simulink model "ultra"  (R2020b)
settings: Solver=FixedStepDiscrete  StartTime=0.0  StopTime=10.0  FixedStep=0.0005  RelTol=1e-3  EnableMultiTasking=on
undefined symbols (not defined in the file): acc_calmax1, acc_calmax2, acc_calmin1, acc_calmin2, akemancanshu, bre, bre_calmax, bre_calmin, ecucoder_acal, I_AN01_5K1, I_AN03_5V, I_AN04_5V, kd, ki, kp, leftmax, O_SW06_HS1A, rightmax, T_add, T_del, tiaoshi, zhiling
libraries: ec5744lib x215, canmsglib x75, simulink x10
(part 6 of 7)

== matlab function ultra/转向自动标定/MATLAB Function1 ==
  data: model input; y output; status input
function y = fcn(model,status)
if (model==2)
    y=1;
else
    y=0;
end

== matlab function ultra/转向自动标定/转向自动标定/MATLAB Function ==
  data: biaozhi1 output
function biaozhi1  = fcn()
persistent i;
     % 初始化状态变量
    if isempty(i)
        i = 1;
    end

    if i>4
        biaozhi1=1;
    else
        biaozhi1=0;       
    end
i=i+1;
end

== matlab function ultra/转向自动标定/转向自动标定/MATLAB Function1 ==
  data: y1 output; y2 output; biaozhi2 output
function [y1,y2,biaozhi2] = fcn()
    persistent i;
     % 初始化状态变量
    if isempty(i)
        i = 1;
    end
    
    if i<4
        biaozhi2=1;
    else
        biaozhi2=0;
    end
    if mod(i, 2) == 0
        result = 1;
    else
        result = 0;
    end
    
    if result==0
        y1=6307883;
        y2=0;
    else
        y1=6307883;
        y2=128;
    end
    i=i+1;

== matlab function ultra/TOWORKSTATION/MATLAB Function ==
  data: u input; y output
function y = fcn(u)
if u~=0&&u~=9&&u~=2
    y=1;
else
    y=0;
end

== matlab function ultra/esc,ABS/Subsystem/MATLAB Function ==
  data: u input; y output; status input
function y = fcn(u,status)
y = u;
if status==5
    u=4500;
end

== matlab function ultra/run/analog_input/有人/Subsystem/MATLAB Function5 ==
  data: acc_fin_sig1 input; y output; acc_fin_sig2 input; bre_ori_sig input; bre input
function y = fcn(acc_fin_sig1, acc_fin_sig2,bre_ori_sig,bre)
if abs(acc_fin_sig1-acc_fin_sig2)>0.6
    y=0;
elseif acc_fin_sig2>0.5&&bre_ori_sig+bre==2
    y=0;
else
    y=acc_fin_sig1;
end

== matlab function ultra/esc,ABS/Subsystem/MATLAB Function1 ==
  data: u input; y output; status input
function y = fcn(u,status)
y = u;
if status==5
    u=4500;
end

== matlab function ultra/esc,ABS/Subsystem/MATLAB Function2 ==
  data: u input; y output; status input
function y = fcn(u,status)
y = u;
if status==5
    u=4500;
end

== matlab function ultra/esc,ABS/Subsystem/MATLAB Function3 ==
  data: u input; y output; status input
function y = fcn(u,status)
y = u;
if status==5
    u=4500;
end

== matlab function ultra/转向自动标定/转向自动标定/Subsystem/MATLAB Function ==
  data: steer output; y output; rm input; lm input; bianmaqi input; k output; d output
function [steer,y,k,d] = fcn(rm,lm,bianmaqi)
%使用前请将转向打到最左侧
lm=lm+3000;
rm=rm-3000;
k=0;
d=0;
  persistent i  A B;
     % 初始化状态变量
    if isempty(i)
        i = 0;
        A=zeros(120,1);
        B=zeros(120,1);
    end
 
    if i>20&&i<=140  
        j=i-20;
        delta=(rm-lm)/120;
        steer= lm+j*delta ;
        if (j>=1&&j<=120)
            B(j,1)=steer-delta;
            A(j,1)=bianmaqi;
        end
        
    else
      if i>=140
            N=length(A);
%             bb=0;
%             aa=0;
%             for l=1:120
%                 bbb=bb+B(l,1);
%                 aaa=aa+A(l,1);
%             end
%             bbar=bbb/120;
%             abar=aaa/120;
            k=(sum(B.*A)-N*mean(B)*mean(A))/(sum(A.^2)-N*mean(A)^2);
            d=mean(B)-k*mean(A);
%             steer=single(d);
        end
        steer=lm;
    end

    i=i+1;
  persistent time  a b;
     % 初始化状态变量
    if isempty(time)
        time = 0;
   
        a=5;
        b=10;
    end
    if mod(abs(time), 2) == 0
        result = 1;
    else
        result = 0;
    end
    if time<b&&result==0
    y=6;
 
    elseif time<b&&result==1
    y=15;
  
    elseif time>=b
        if result==1
            y=79;
        else
            y=63;
        end
    else
        y=6;
    end   
    time=time+1;
 
%     
%       persistent time1;
%      % 初始化状态变量
%     if isempty(time1)
%         time1 = 0;
%     end
%     if mod(time1, 2) == 0
%         result1 = 1;
%     else
%         result1 = 0;
%     end
%     if time1<2
%     y=6;
%  
%     elseif time1>=2&&time1<4
%     y=15;
%   
%     elseif time1>=4
%         if result1==1
%             y=79;
%         else
%             y=63;
%         end
%     else
%         y=6;
%     end   
%     time1=time1+1;
   
end

== matlab function ultra/run/analog_input/有人/Subsystem/Subsystem1/MATLAB Function ==
  data: u input; y output
function y = fcn(u)
if u==0
    y=0;
else
    y=1;
end

== matlab function ultra/run/MATLAB Function ==
  data: u input; y output; u1 input; model input
function y = fcn(u,u1,model)
if ((u>0.8&&model==0)||(u1>0.8))
    y = 1;
else
    y=0;
end

== matlab function ultra/run/LQR ==
  data: x input; y output
function y = fcn(x)
% A=[1 1;1 1];
% size(A,1);
% B=[1;1];
% P=size(B,2);
% ts=0.02;%离散时间的步长
% sys_d=c2d(ss(A,B),ts);%连续转离散系统函数，用于仿真代码
% x0=[1,1];%系统初始化
% x=x0;
% u0=0;
% u=u0;
% Q=[1 0 ;0 1];%系统权重
% S=[1 0;0 1];%终值权重
% R=0.1;%输入权重
% %定义系统运行步数
% k_steps = 100;
% %定义x._history雩矩阵,用于储存系统状态结果
% xhistory = zeros(n ,k_steps) ;
% %俘系统状态初始值赋值到x_history矩阵第一个位置
% xhistory (:,l)= x;
% %定义u_history需矩阵,用于储存系统输入结果,
% u_history = zeros(p,k_steps) ;
% %俘系统输入初始值赋值到u_history矩阵第一个位置
% u_history (:,1) = u;
% P_k = s;
% %计算最优反馈增益
% 
% 
% % 计算最优反馈增益
% for k = l : N
% % 计算F[N-k]
% F= inv(R+B'*P_k*B)*B'*P_k*A;
% 
% N= k_steps;
% P_k = s;
% % 计算最优反馈增益
% 
% P_k = (A-B*F)'*P_k*(A-B*F)+(F)'*R*(F)+Q;
% if k ==l
% F_N=F;
% else
% F_N=[F;F_N];
% end
% %仿真开始,建立for循环
% for k=l:k_steps
% u =-FN((k-1)*p+l:k*p ,:)*x;
% x= A*x+B*u ;
% %保存系统状态到预先定义矩阵的相应位置
% x_history(: ,k+l)=x;
% %保存系统输入到预先定义矩阵的相应位置
% u_history ( :,k)=u ;
% end
% 
% y=u;

== matlab function ultra/run/ctrl/Subsystem1/control_strategy/MPC ==
  data: X_K input; y output; Prediction input; A input; B input; Q input; R input; F input
function y = fcn(X_K,Prediction,A,B,Q,R,F)
    U_K(:,k) = Prediction;
    % 计算第k+1步时状态变量的值
%     X_K(:,k+1) = (A*X_K(:,k) + B*U_K(:,k))-0.17*A;
end

== matlab function ultra/run/ctrl/Subsystem1/control_strategy/限滑/MPC/MPC/MPC右后/MPC_function ==
  data: x_k input; u_k output; U_init input
function u_k= Prediction(x_k,U_init)
% 定义状态矩阵 A, n*n 矩阵
A = 0;
% 定义输入矩阵 B, n*p 矩阵
R=0.2032;
FN=2058;
K=6.89;
B = R/(FN*K);
p = size(B,2);
% 定义Q矩阵，n*n 矩阵
Q = 100;
% 定义F矩阵，n*n 矩阵
F = 100;
% 定义R矩阵，p*p 矩阵
R = 1;
% 定义迭代次数和学习率
maxIterations = 5;
learningRate = 0.3;
N=5;%预测区间
n=size(A,1); % A是n*n矩阵,得到n
p=size(B,2); % B是n*p矩阵,得到p
M=[eye(n);zeros(N*n,n)]; % 初始化M矩阵,M矩阵是(N+1)n*n的
D=[0.17;zeros(N*n,n)];
C=zeros((N+1)*n,N*p); % 初始化C矩阵,这一步令它有(N+1)n*NP个0

% 定义M和C
tmp=eye(n); % 定义一个n*n 的 I 矩阵
    for i=1:N % 循环,i从1到N
        rows =i*n+(1:n); %定义当前行数,从i*n开始，共n行
        C(rows,:)=[tmp*B,C(rows-n, 1:end-p)]; %将c矩阵填满
        tmp= A*tmp; %每一次将tmp左乘一次A
        M(rows,:)=tmp; %将M矩阵写满
         D(rows,:)=0.17;
    end
    % 定义Q_bar和R_bar
    Q_bar = kron(eye(N),Q);
    Q_bar = blkdiag(Q_bar,F);
    R_bar = kron(eye(N),R);
    % 计算G,E,H
    G=M'*Q_bar*M; % G: n*n
    E=C'*Q_bar*M; % E: NP*n
    H=C'*Q_bar*C+R_bar; % NP*NP
 J=(D'*Q_bar*C)';
 L=E*x_k+J;
 U = U_init*ones(N*p,1); % NP x 1
%  options = optimoptions('quadprog', 'Algorithm', 'active-set');
%  U_k = quadprog(H,L, [], [], [], [], 0*ones(5,1), 1100*ones(5,1), 100*ones(5,1), options);
    % 梯度下降法求解最优二次规划问题
    G=size(U,1);
    S=zeros(G*maxIterations,1);
    for i = 1:maxIterations
        % 计算目标函数的梯度
        gradient = 2*H*U + 2*L;
        % 更新变量 U，并保持在 [0, 1100] 范围内
        U = U - learningRate * gradient;
        U = max(U, 0);
        U = min(U, 1100);
        O=(i-1)*maxIterations+(1:maxIterations);
        S(O,1)=U;
    end

 u_k = S(1:p,1); % 取第一个结果
end

== matlab function ultra/run/ctrl/Subsystem1/control_strategy/E,H ==
  data: A input; E output; B input; Q input; R input; F input; N input; H output; J output
function [E,H,J] = MPC_Matrices(A,B,Q,R,F,N)
    n=size(A,1); % A是n*n矩阵,得到n
    p=size(B,2); % B是n*p矩阵,得到p
    M=[eye(n);zeros(N*n,n)]; % 初始化M矩阵,M矩阵是(N+1)n*n的,
                             % 它上面是n*n个"I",这一步先把下半部分写成0
    C=zeros((N+1)*n,N*p); % 初始化C矩阵,这一步令它有(N+1)n*NP个0
     D=zeros(1,N*p);
    % 定义M和C
    tmp=eye(n); % 定义一个n*n 的 I 矩阵
    % 更新Ｍ和C
    for i=1:N % 循环,i从1到N
        rows =i*n+(1:n); %定义当前行数,从i*n开始，共n行
        C(rows,:)=[tmp*B,C(rows-n, 1:end-p)]; %将c矩阵填满
        tmp= A*tmp; %每一次将tmp左乘一次A
        M(rows,:)=tmp; %将M矩阵写满
    end
    % 定义Q_bar和R_bar
    Q_bar = kron(eye(N),Q);
    Q_bar = blkdiag(Q_bar,F);
    R_bar = kron(eye(N),R);
    % 计算G,E,H
    G=M'*Q_bar*M; % G: n*n
    E=C'*Q_bar*M; % E: NP*n
    H=C'*Q_bar*C+R_bar; % NP*NP
for i=1:N % 循环,i从1到N
     D(i)= 0.17;
end
  J=C'*Q_bar*D'

== matlab function ultra/run/ctrl/Subsystem1/control_strategy/MATLAB Function2 ==
  data: A output; B output; Q output; R output; F output; N output; p output
function [A,B,Q,R,F,N,p] = fcn()
% 定义状态矩阵 A, n*n 矩阵
A = 0;
% 定义输入矩阵 B, n*p 矩阵
R=1;
FN=1;
K=6.89;
B = R/(FN*K);
p = size(B,2);
% 定义Q矩阵，n*n 矩阵
Q = 100;
% 定义F矩阵，n*n 矩阵
F = 100;
% 定义R矩阵，p*p 矩阵
R = 1;
%定义预测区间K
N = 5;

== matlab function ultra/run/ctrl/Subsystem1/control_strategy/差速/差速/LQR差速 ==
  data: yaw_error input; M output; yaw_rate input; J input
% function M = carLQRControl(yaw_error, yaw_rate,J)
%     % 赛车LQR控制器参数
%     Q = diag([1, 1]); % 状态误差权重矩阵
%     R = 0.1; % 控制输入权重
%     
%     % 定义车辆模型参数
%     % J转动惯量
%     
%     % 设计LQR增益矩阵 K
%     A = [0, 1; 0, 0];%输入为期望与实际横摆力矩差值和横摆角速度
%     B = [0; J];
%     K = lqr(A, B, Q, R);
%     
%     % 计算横摆力矩控制输入
%     M = -K* [yaw_error; yaw_rate];
function M = carLQRControl(yaw_error, yaw_rate,J)
    % 赛车LQR控制器参数
    Q = diag([1, 1]); % 状态误差权重矩阵
    R = 0.1; % 控制输入权重
    
    % 设计LQR增益矩阵 K
    A = [0, 1; 0, 0]; % 输入为期望与实际横摆力矩差值和横摆角速度
    B = [0; J];
    
    % 使用迭代法求解代数Riccati方程，计算LQR增益矩阵 K
    max_iterations = 20;
    tolerance = 1e-2;
    P = eye(size(A));
%     for i = 1:max_iterations
%         P_new = Q + A' * P * A - A' * P * B * (R + B' * P * B)^(-1) * B' * P * A;
%         if max(abs(P_new - P), [], 'all') < tolerance
%             P = P_new;
%             break;
%         end
%         P = P_new;
%   K = (R + B' * P * B)^(-1) * B' * P * A;
%     end
     % 计算LQR增益矩阵 

 
   for k = 1:max_iterations
        F = inv(R+B'*P*B)*B'*P*A;
        P_new = (A-B*F)'*P*(A-B*F)+(F)'*R*(F)+Q;
        if max(abs(P_new - P), [], 'all') < tolerance
             P= P_new;
             F = inv(R+B'*P*B)*B'*P*A;
            break;
        end
        P= P_new;
    end
    F_N=F; 
   
    % 计算横摆力矩控制输入
    M = -F_N * [yaw_error; yaw_rate];

end

== matlab function ultra/run/ctrl/Subsystem1/control_strategy/限滑/MPC/MPC/MPC左后/MPC_function ==
  data: x_k input; u_k output; U_init input
function u_k= Prediction(x_k,U_init)
% 定义状态矩阵 A, n*n 矩阵
A = 0;
% 定义输入矩阵 B, n*p 矩阵
R=0.2032;
FN=2058;
K=6.89;
B = R/(FN*K);
p = size(B,2);
% 定义Q矩阵，n*n 矩阵
Q = 100;
% 定义F矩阵，n*n 矩阵
F = 100;
% 定义R矩阵，p*p 矩阵
R = 1;
% 定义迭代次数和学习率
maxIterations = 5;
learningRate = 0.3;
N=5;%预测区间
n=size(A,1); % A是n*n矩阵,得到n
p=size(B,2); % B是n*p矩阵,得到p
M=[eye(n);zeros(N*n,n)]; % 初始化M矩阵,M矩阵是(N+1)n*n的
D=[0.17;zeros(N*n,n)];
C=zeros((N+1)*n,N*p); % 初始化C矩阵,这一步令它有(N+1)n*NP个0

% 定义M和C
tmp=eye(n); % 定义一个n*n 的 I 矩阵
    for i=1:N % 循环,i从1到N
        rows =i*n+(1:n); %定义当前行数,从i*n开始，共n行
        C(rows,:)=[tmp*B,C(rows-n, 1:end-p)]; %将c矩阵填满
        tmp= A*tmp; %每一次将tmp左乘一次A
        M(rows,:)=tmp; %将M矩阵写满
         D(rows,:)=0.17;
    end
    % 定义Q_bar和R_bar
    Q_bar = kron(eye(N),Q);
    Q_bar = blkdiag(Q_bar,F);
    R_bar = kron(eye(N),R);
    % 计算G,E,H
    G=M'*Q_bar*M; % G: n*n
    E=C'*Q_bar*M; % E: NP*n
    H=C'*Q_bar*C+R_bar; % NP*NP
 J=(D'*Q_bar*C)';
 L=E*x_k+J;
 U = U_init*ones(N*p,1); % NP x 1
%  options = optimoptions('quadprog', 'Algorithm', 'active-set');
%  U_k = quadprog(H,L, [], [], [], [], 0*ones(5,1), 1100*ones(5,1), 100*ones(5,1), options);
    % 梯度下降法求解最优二次规划问题
    G=size(U,1);
    S=zeros(G*maxIterations,1);
    for i = 1:maxIterations
        % 计算目标函数的梯度
        gradient = 2*H*U + 2*L;
        % 更新变量 U，并保持在 [0, 1100] 范围内
        U = U - learningRate * gradient;
        U = max(U, 0);
        U = min(U, 1100);
        O=(i-1)*maxIterations+(1:maxIterations);
        S(O,1)=U;
    end

 u_k = S(1:p,1); % 取第一个结果
end

== matlab function ultra/run/ctrl/Subsystem1/control_strategy/限滑/MPC/MPC/MPC右前/MPC_function ==
  data: x_k input; u_k output; U_init input
function u_k= Prediction(x_k,U_init)
% 定义状态矩阵 A, n*n 矩阵
A = 0;
% 定义输入矩阵 B, n*p 矩阵
R=0.2032;
FN=2058;
K=6.89;
B = R/(FN*K);
p = size(B,2);
% 定义Q矩阵，n*n 矩阵
Q = 100;
% 定义F矩阵，n*n 矩阵
F = 100;
% 定义R矩阵，p*p 矩阵
R = 1;
% 定义迭代次数和学习率
maxIterations = 5;
learningRate = 0.3;
N=5;%预测区间
n=size(A,1); % A是n*n矩阵,得到n
p=size(B,2); % B是n*p矩阵,得到p
M=[eye(n);zeros(N*n,n)]; % 初始化M矩阵,M矩阵是(N+1)n*n的
D=[0.17;zeros(N*n,n)];
C=zeros((N+1)*n,N*p); % 初始化C矩阵,这一步令它有(N+1)n*NP个0

% 定义M和C
tmp=eye(n); % 定义一个n*n 的 I 矩阵
    for i=1:N % 循环,i从1到N
        rows =i*n+(1:n); %定义当前行数,从i*n开始，共n行
        C(rows,:)=[tmp*B,C(rows-n, 1:end-p)]; %将c矩阵填满
        tmp= A*tmp; %每一次将tmp左乘一次A
        M(rows,:)=tmp; %将M矩阵写满
         D(rows,:)=0.17;
    end
    % 定义Q_bar和R_bar
    Q_bar = kron(eye(N),Q);
    Q_bar = blkdiag(Q_bar,F);
    R_bar = kron(eye(N),R);
    % 计算G,E,H
    G=M'*Q_bar*M; % G: n*n
    E=C'*Q_bar*M; % E: NP*n
    H=C'*Q_bar*C+R_bar; % NP*NP
 J=(D'*Q_bar*C)';
 L=E*x_k+J;
 U = U_init*ones(N*p,1); % NP x 1
%  options = optimoptions('quadprog', 'Algorithm', 'active-set');
%  U_k = quadprog(H,L, [], [], [], [], 0*ones(5,1), 1100*ones(5,1), 100*ones(5,1), options);
    % 梯度下降法求解最优二次规划问题
    G=size(U,1);
    S=zeros(G*maxIterations,1);
    for i = 1:maxIterations
        % 计算目标函数的梯度
        gradient = 2*H*U + 2*L;
        % 更新变量 U，并保持在 [0, 1100] 范围内
        U = U - learningRate * gradient;
        U = max(U, 0);
        U = min(U, 1100);
        O=(i-1)*maxIterations+(1:maxIterations);
        S(O,1)=U;
    end

 u_k = S(1:p,1); % 取第一个结果
end

== matlab function ultra/run/ctrl/Subsystem1/control_strategy/限滑/MPC/MPC/MPC左前/MPC_function ==
  data: x_k input; u_k output; U_init input
function u_k= Prediction(x_k,U_init)
% 定义状态矩阵 A, n*n 矩阵
A = 0;
% 定义输入矩阵 B, n*p 矩阵
R=0.2032;
FN=2058;
K=6.89;
B = R/(FN*K);
p = size(B,2);
% 定义Q矩阵，n*n 矩阵
Q = 100;
% 定义F矩阵，n*n 矩阵
F = 100;
% 定义R矩阵，p*p 矩阵
R = 1;
% 定义迭代次数和学习率
maxIterations = 5;
learningRate = 0.3;
N=5;%预测区间
n=size(A,1); % A是n*n矩阵,得到n
p=size(B,2); % B是n*p矩阵,得到p
M=[eye(n);zeros(N*n,n)]; % 初始化M矩阵,M矩阵是(N+1)n*n的
D=[0.17;zeros(N*n,n)];
C=zeros((N+1)*n,N*p); % 初始化C矩阵,这一步令它有(N+1)n*NP个0

% 定义M和C
tmp=eye(n); % 定义一个n*n 的 I 矩阵
    for i=1:N % 循环,i从1到N
        rows =i*n+(1:n); %定义当前行数,从i*n开始，共n行
        C(rows,:)=[tmp*B,C(rows-n, 1:end-p)]; %将c矩阵填满
        tmp= A*tmp; %每一次将tmp左乘一次A
        M(rows,:)=tmp; %将M矩阵写满
         D(rows,:)=0.17;
    end
    % 定义Q_bar和R_bar
    Q_bar = kron(eye(N),Q);
    Q_bar = blkdiag(Q_bar,F);
    R_bar = kron(eye(N),R);
    % 计算G,E,H
    G=M'*Q_bar*M; % G: n*n
    E=C'*Q_bar*M; % E: NP*n
    H=C'*Q_bar*C+R_bar; % NP*NP
 J=(D'*Q_bar*C)';
 L=E*x_k+J;
 U = U_init*ones(N*p,1); % NP x 1
%  options = optimoptions('quadprog', 'Algorithm', 'active-set');
%  U_k = quadprog(H,L, [], [], [], [], 0*ones(5,1), 1100*ones(5,1), 100*ones(5,1), options);
    % 梯度下降法求解最优二次规划问题
    G=size(U,1);
    S=zeros(G*maxIterations,1);
    for i = 1:maxIterations
        % 计算目标函数的梯度
        gradient = 2*H*U + 2*L;
        % 更新变量 U，并保持在 [0, 1100] 范围内
        U = U - learningRate * gradient;
        U = max(U, 0);
        U = min(U, 1100);
        O=(i-1)*maxIterations+(1:maxIterations);
        S(O,1)=U;
    end

 u_k = S(1:p,1); % 取第一个结果
end

== matlab function ultra/run/ctrl/Subsystem1/control_strategy/限滑/PID限滑/pid限滑与ABS ==
  data: slip input; throttle output; slip_ratio_limit input; brake output; u input
function [throttle, brake] = carPIDWithSlipControl(slip, slip_ratio_limit,u)
    % 赛车PID控制器参数
    kp = 0.2;
    ki = 0.1;
    kd = 0.01;
    
    % 状态变量
    persistent integral previous_error i
    
    % 初始化状态变量
    if isempty(integral)
        integral = 0;
        previous_error = 0;
        i=0;
    end
    
    % PID控制器计算
    error = 0.2 - slip;
    integral = integral + error*0.02;
    derivative = (error - previous_error)/0.02;
    
   k = kp * error + ki * integral + kd * derivative;
    if i<100
    
        output = u+k*u;
        if output>2000
            output=2000;
        end
    else
        output=u;
    end
    % 根据滑移率限制输出
  
    if slip > slip_ratio_limit
        brake = 0;%output;
        throttle = 0;
    else
        brake = 0;
        throttle = output;
    end
    
    % 保存上一个误差用于下次计算
    previous_error = error;

    i=i+1;
end

== matlab function ultra/run/analog_input/无人意图转译/无人/Subsystem1/MATLAB Function3 ==
  data: u input; y1 output; y2 output; v input; vd input; ade input; adede input; adedede input
function [y1,y2] = fcn(u,v,vd,ade,adede,adedede)
persistent i
    if isempty(i)
       
        i=0;
    end
dota=(u-i);
if v-vd>5
    u=0;
end
if u>=0
    if dota>1
    y1=(u+i+ade+adede+adedede)/5;
    else
    y1=u;
    end
    y2=0;
else
    y1=0;
    y2=u;
end

if u<0
    y2=u;
end
i=u;
end

== matlab function ultra/run/analog_input/无人意图转译/无人/Subsystem1/Subsystem/pid_function/integral ==
  data: u input; output output; a input
function output = fcn(u,a)
    % 赛车PID控制器参数
    kp = 0;
    ki = 0;
    kd = 0;
    
    % 状态变量
    persistent integral previous_error i
    
    % 初始化状态变量
    if isempty(integral)
        integral = 0;
        previous_error = 0;
        i=0;
    end
        if i>50
            i=0;
            ki = 0;
            kd = 0;
        end
    % PID控制器计算
    error = u;
%     integral = integral + error*0.02;
    derivative = (error - previous_error)/0.02;
    integral =0;
    if error<0.1
        ki=0;
    end
    output = kp * error + ki * integral + kd * derivative;
    
   if a==0
       output=0;
   end
    % 保存上一个误差用于下次计算
    previous_error = error;
    i=i+1
end

== matlab function ultra/run/analog_input/有人/Subsystem/MATLAB Function1 ==
  data: u input; y output; min input; max input
function y = fcn(u,min,max)
% 
% y = (double(u)-min-1270)/(max-min+2980-1270);
% y=0;
y=u;

== matlab function ultra/run/analog_input/无人意图转译/无人/Subsystem1/计算四轮各自制动力/MATLAB Function ==
  data: u input; y1 output; y2 output; y3 output; y4 output; deltaM input
function [y1,y2,y3,y4] = fcn(u,deltaM)


deltaM=0;
B=1.17;%轮距,前轮1.18后轮1.16
F1=1050;
F2=1050;%前后轮载荷，瞎设的，合并后引入
%a1 a2 b1 b2分别是左前轮制动力，右前轮制动力，左后轮制动力，右后轮制动力 方程： a1+a2+b1+b2==u/r;(a1+a2)/F1==(b1+b2)/F2;B*(a1-a2)/(2*F1)==B*(b1-b2)/(2*F2);(a1-a2)*B/2+(b1-b2)*B/2==deltaM;
b1=F2*u/(2*(F1+F2))+F2*deltaM/(F1*B+F2*B);
b2=F2*u/(2*(F1+F2))-F2*deltaM/(F1*B+F2*B);
a1=u/2-F2*u/(2*(F1+F2))+F1*deltaM/(F1*B+F2*B);
a2=u/2-F2*u/(2*(F1+F2))-F1*deltaM/(F1*B+F2*B);
y1=a1;
y2=a2;
y3=b1;
y4=b2;

== matlab function ultra/run/analog_input/无人意图转译/无人/Subsystem1/计算油压 ==
  data: y1 input; p1 output; y2 input; y3 input; y4 input; p2 output; p3 output; p4 output; zuoqian input; youqian input; zuohou input; youhou input; error input
function [p1,p2,p3,p4]= fcn(y1,y2,y3,y4,zuoqian,youqian,zuohou,youhou,error)
S=0.000491;
%p1 p2 p3 p4分别是左前、右前、左后、右后油压
p1=y1/(0.8*S)/1000*1.2;
p2=y2/(0.8*S)/1000*1.2;
p3=y3/(0.4*S)/1000*0.8;
p4=y4/(0.4*S)/1000*0.8;
    % 状态变量
    persistent  i1 i2 i3 i4 pp1 pp2 pp3 pp4
    
    % 初始化状态变量
    if isempty(i1)
        i1=0;
        i2=0;
        i3=0;
        i4=0;
        pp1=0;
        pp2=0;
        pp3=0;
        pp4=0;
    end
if abs(error)>0.6
    if p1>500||i1>0
        i1=i1+1;
        if p1<pp1
            if pp1-zuoqian>300
                p1=pp1-20;
            end
        end
    end
    if i1>49||abs(p1-zuoqian)<200
        i1=0;
    end
    if p2>500||i2>0
        i2=i2+1;
        if p2<pp2
            if pp2-youqian>300
                p2=pp2-20;
            end
        end
    end
    if i2>49||abs(p2-youqian)<200
        i2=0;
    end
    if p3>500||i3>0
        i3=i3+1;
        if p3<pp3
            if pp3-zuohou>300
                p3=pp3-20;
            end
        end
    end
    if i3>49||abs(p3-zuohou)<200
        i3=0;
    end
    if p4>500||i4>0
        i4=i4+1;
        if p4<pp4
            if pp4-youhou>300
                p4=pp4-20;
            end
        end
    end
    if i4>49||abs(p4-youhou)<200
        i4=0;
    end
end
 if error>0
     p1=0;
     p2=0;
     p3=0;
     p4=0;
 end
    pp1=p1;
    pp2=p2;
    pp3=p3;
    pp4=p4;
 
% if p1<0
%     p1=0;
%     end
% if p2<0
%     p2=0;
%     end
% if p3<0
%     p3=0;
%     end
% if p4<0
%     p4=0;
% end

== matlab function ultra/run/analog_input/无人意图转译/无人/MATLAB Function3 ==
  data: u input; y output
function y = fcn(u)
if u~=0
    y = 1;
else
    y=0;
end

== matlab function ultra/run/analog_input/无人意图转译/计算期望扭矩 ==
  data: u input; y output; canok input
function y = fcn(u,canok)

y = u*230*86.08;
if y>2000
    y=2000;
end
if canok==0
    y=0;
end

== matlab function ultra/run/analog_input/无人意图转译/无人/Subsystem1/id ==
  data: u input; output output
function output = fcn(u)
    % 赛车ID控制器参数
  
    ki = 0;
    kd = 0;
    
    % 状态变量
    persistent integral previous_error i
    
    % 初始化状态变量
    if isempty(integral)
        integral = 0;
        previous_error = 0;
        i=0;
    end
    if i>50
        i=0;
        ki = 0;
        kd = 0;
    end
    % PID控制器计算
    error = u;
    integral = integral + error*0.02;
    derivative = (error - previous_error)/0.02;
     if error<0.1
        ki=0;
    end
    output =  ki * integral + kd * derivative;
    if error<0.1
        ki=0;
    end
  
    % 保存上一个误差用于下次计算
    previous_error = error;
    if output>10
        output=0;
    end
    i=i+1;
end

== matlab function ultra/RX/lcu——receive/Subsystem1/Subsystem/MATLAB Function ==
  data: m input; y1 output; y2 output; y3 output
function [y1,y2,y3] = fcn(m)
V=zeros(1,3);
a=2;i=3;
while i>0
    V(1,i)=mod(m,a);
    m=fix(m/2);
    i=i-1;
end  
y1 = V(1,3);
y2=V(1,2);
y3=V(1,1);
end

== matlab function ultra/RX/lcu——receive/Subsystem1/Subsystem/MATLAB Function1 ==
  data: u input; y output
function y = fcn(u)
if u==7
    y = 1;
else
    y=0;
end
end

== matlab function ultra/run/ctrl/Subsystem1/control_strategy/差速/差速/期望横摆力矩计算 ==
  data: delta input; Mz output; Vx input; ax input
function Mz = calculateYawMoment(delta,  Vx, ax)
    % 输入参数：
    % delta: 前轮转角 (rad)
    % Vx: 车辆速度 (m/s)
    % ax: 侧向加速度 (m/s^2)
    m=210;%: 车辆质量 (kg)
     lf=0.765;%: 前轴到重心的距离 (m)
     lr=0.765;%: 后轴到重心的距离 (m)
    
    % 轮胎侧向力估计，这里使用一个简化的线性模型
    Fy = ax * (lr * m * 9.81) / (lf + lr);
    delta=delta*pi/180
    % 计算期望的横摆力矩
    Mz = lf * Fy * cos(delta);
end

== matlab function ultra/run/ctrl/Subsystem1/control_strategy/限滑/PID限滑/pid限滑与ABS1 ==
  data: slip input; throttle output; slip_ratio_limit input; brake output; u input
function [throttle, brake] = carPIDWithSlipControl(slip, slip_ratio_limit,u)
    % 赛车PID控制器参数
    kp = 0.2;
    ki = 0.1;
    kd = 0.01;
    
    % 状态变量
    persistent integral previous_error i
    
    % 初始化状态变量
    if isempty(integral)
        integral = 0;
        previous_error = 0;
        i=0;
    end
    
    % PID控制器计算
    error = 0.2 - slip;
    integral = integral + error*0.02;
    derivative = (error - previous_error)/0.02;
    
   k = kp * error + ki * integral + kd * derivative;
    if i<100
    
        output = u+k*u;
        if output>2000
            output=2000;
        end
    else
        output=u;
    end
    % 根据滑移率限制输出
  
    if slip > slip_ratio_limit
        brake = 0;%output;
        throttle = 0;
    else
        brake = 0;
        throttle = output;
    end
    
    % 保存上一个误差用于下次计算
    previous_error = error;
    i=i+1;
end

== matlab function ultra/run/analog_input/有人/Subsystem/MATLAB Function ==
  data: u input; y output; min input; max input
function y = fcn(u,min,max)

y = (double(u)-min-4765)/(-min+max-4765+4900);

== matlab function ultra/run/ctrl/Subsystem1/control_strategy/限滑/PID限滑/pid限滑与ABS2 ==
  data: slip input; throttle output; slip_ratio_limit input; brake output; u input
function [throttle, brake] = carPIDWithSlipControl(slip, slip_ratio_limit,u)
    % 赛车PID控制器参数
    kp = 0.2;
    ki = 0.1;
    kd = 0.01;
    
    % 状态变量
    persistent integral previous_error i
    
    % 初始化状态变量
    if isempty(integral)
        integral = 0;
        previous_error = 0;
        i=0;
    end
    
    % PID控制器计算
    error = 0.2 - slip;
    integral = integral + error*0.02;
    derivative = (error - previous_error)/0.02;
   k = kp * error + ki * integral + kd * derivative;
    if i<100
    
        output = u+k*u;
        if output>2000
            output=2000;
        end
    else
        output=u;
    end
    % 根据滑移率限制输出
  
    if slip > slip_ratio_limit
        brake = 0;%output;
        throttle = 0;
    else
        brake = 0;
        throttle = output;
    end
    
    % 保存上一个误差用于下次计算
    previous_error = error;
    i=i+1;
end

== matlab function ultra/run/ctrl/Subsystem1/control_strategy/限滑/PID限滑/pid限滑与ABS3 ==
  data: slip input; throttle output; slip_ratio_limit input; brake output; u input
function [throttle, brake] = carPIDWithSlipControl(slip, slip_ratio_limit,u)
    % 赛车PID控制器参数
    kp = 0.2;
    ki = 0.1;
    kd = 0.01;
    
    % 状态变量
    persistent integral previous_error i
    
    % 初始化状态变量
    if isempty(integral)
        integral = 0;
        previous_error = 0;
        i=0;
    end
    
    % PID控制器计算
    error = 0.2 - slip;
    integral = integral + error*0.02;
    derivative = (error - previous_error)/0.02;
    
   k = kp * error + ki * integral + kd * derivative;
    if i<100
    
        output = u+k*u;
        if output>2000
            output=2000;
        end
    else
        output=u;
    end
    % 根据滑移率限制输出
  
    if slip > slip_ratio_limit
        brake =0;% output;
        throttle = 0;
    else
        brake = 0;
        throttle = output;
    end
    
    % 保存上一个误差用于下次计算
    previous_error = error;
    i=i+1;
end

== matlab function ultra/run/ctrl/Subsystem1/control_strategy/MATLAB Function1 ==
  data: y output; angle input
function y = fcn(angle)
if angle>30||angle<-30%4650000,4870000,4741002
    y=1;
else
    y = 0;
end

== matlab function ultra/run/ctrl/Subsystem1/control_strategy/限滑/Subsystem1/MATLAB Function2 ==
  data: u input; y output; mpc input; pid input; slip input; model input
function y = fcn(u,mpc,pid,slip,model)
if slip>0.8&&model~=6
    y=pid;
elseif slip>0.165&&slip<0.17
        y=mpc;
else
        y=u;
end
end

== matlab function ultra/run/ctrl/Subsystem1/control_strategy/限滑/Subsystem1/MATLAB Function3 ==
  data: u input; y output; mpc input; pid input; slip input; model input
function y = fcn(u,mpc,pid,slip,model)
if slip>0.8&&model~=6
    y=pid;
elseif slip>0.169&&slip<0.17
        y=mpc;
else
        y=u;
end
end

== matlab function ultra/run/ctrl/Subsystem1/control_strategy/限滑/Subsystem1/MATLAB Function4 ==
  data: u input; y output; mpc input; pid input; slip input; model input
function y = fcn(u,mpc,pid,slip,model)
if slip>0.8&&model~=6
    y=pid;
elseif slip>0.165&&slip<0.17
        y=mpc;
else
        y=u;
end
end

== matlab function ultra/run/ctrl/Subsystem1/control_strategy/限滑/Subsystem1/MATLAB Function5 ==
  data: u input; y output; mpc input; pid input; slip input; model input
function y = fcn(u,mpc,pid,slip,model)
if slip>0.8&&model~=6
    y=pid;
elseif slip>0.165&&slip<0.17
        y=mpc;
else
        y=u;
end
end

== matlab function ultra/run/ctrl/Subsystem1/control_strategy/差速/MATLAB Function3 ==
  data: u input; youhou output; M input; youqian output; zuohou output; zuoqian output
function [youhou,youqian,zuohou,zuoqian] = fcn(u,M)
% U=4*u;
r=0.2032;%轮半径
B1=1.18;%左右轮距
B2=1.16;
youqian=M*r/(2*B2)+u;
youhou=youqian;
zuoqian=-M*r/(2*B1)+u;
zuohou=zuoqian;
end

== matlab function ultra/run/ctrl/Subsystem1/control_strategy/Subsystem/defuzzification ==
  data: dnb input; delta output; dns input; do input; dps input; dpb input; d1 input; d2 input; d3 input
function delta = fcn(dnb,dns,do,dps,dpb, d1,d2,d3)
delta = dnb*d1/3 + dns*d1 + do*d2 + dps*d3 + dpb*(1-d3/3);
end

== matlab function ultra/run/analog_input/有人/Subsystem/MATLAB Function2 ==
  data: u input; y output; min input; max input
function y = fcn(u,min,max)

y = (double(u)-min-4670)/(-min+0.01+max-4670+4550);

== matlab function ultra/run/ctrl/Subsystem1/control_strategy/Subsystem/α sets ==
  data: alpha input; as output; am output; ab output; a1 input; a2 input
function [as,am,ab] = fcn(alpha, a1, a2)
if alpha < a1
    as = 1-(alpha/a1);
    am = alpha/a1;
    ab = 0;
elseif alpha < a2
    as = 0; 
    am = 1-(alpha-a1)/(a2-a1);
    ab = (alpha-a1)/(a2-a1);
else
    as = 0;
    am = 0;
    ab = 1;
end

== matlab function ultra/run/ctrl/Subsystem1/control_strategy/Subsystem/β sets ==
  data: beta input; bnb output; bns output; bo output; b1 input; b2 input; bps output; bpb output; b3 input
function [bnb,bns,bo,bps,bpb] = fcn(beta, b1, b2, b3)
if beta < b1
    bnb = 1-(beta+1)/(b1+1);
    bns = (beta+1)/(b1+1);
    bo  = 0;
    bps = 0;
    bpb = 0;
elseif beta < b2
    bnb = 0; 
    bns = 1-(beta-b1)/(b2-b1);
    bo = (beta-b1)/(b2-b1);
    bps = 0;
    bpb = 0;
elseif beta < b3
    bnb = 0;
    bns = 0;
    bo  = 1-(beta-b2)/(b3-b2);
    bps = (beta-b2)/(b3-b2);
    bpb = 0;
else
    bnb = 0;
    bns = 0;
    bo  = 0;
    bps = 1-(beta-b3)/(1-b3);
    bpb = (beta-b3)/(1-b3);
end

== matlab function ultra/run/ctrl/Subsystem1/control_strategy/限滑/PID限滑/计算油压 ==
  data: y1 input; p1 output; y2 input; y3 input; y4 input; p2 output; p3 output; p4 output
function [p1,p2,p3,p4]= fcn(y1,y2,y3,y4)
S=0.000491;
%p1 p2 p3 p4分别是左前、右前、左后、右后油压
p1=y1/(0.8*S)/1000;
p2=y2/(0.8*S)/1000;
p3=y3/(0.4*S)/1000;
p4=y4/(0.4*S)/1000;
% if p1<0
%     p1=0;
%     end
% if p2<0
%     p2=0;
%     end
% if p3<0
%     p3=0;
%     end
% if p4<0
%     p4=0;
% end

== matlab function ultra/TX控制器/速度/184左前/MATLAB Function1 ==
  data: v input; T output; a input
function T = fcn(v,a)
% if a>5
%     y = u;
% elseif a>3&&a<5
%     y=1200;
% else
%     y=800;
% end

if v<6000*1.88e-3
    T=2100;
elseif v>11000*1.88e-3
    T=800;
else
    T=1100;
end

== matlab function ultra/TX控制器/速度/188右后/MATLAB Function1 ==
  data: v input; T output; a input
function T = fcn(v,a)
% if a>5
%     y = u;
% elseif a>3&&a<5
%     y=1200;
% else
%     y=800;
% end

if v<6000*1.88e-3
    T=2100;
elseif v>11000*1.88e-3
    T=800;
else
    T=1100;
end

== matlab function ultra/RX/转向——receive1/Subsystem3/Subsystem/MATLAB Function ==
  data: u input; y output
function y = fcn(u)
y =   0.0003056 *u-208.4  ;
if u==683198
    y=0;
end

== matlab function ultra/run/analog_input/MATLAB Function2 ==
  data: u input; y output; canok input
function y = fcn(u,canok)
if u==0%&&canok==1
    y=1;
else
    y=0;
end

== matlab function ultra/run/ctrl/Subsystem1/control_strategy/差速/差速/MATLAB Function ==
  data: u input; y output
function y = fcn(u)

y = u;

== matlab function ultra/run/MATLAB Function2 ==
  data: u input; y output
function y = fcn(u)
if u>500
    y=1;
else
    y=0;
end
if u>1800
    y=2;
end

== matlab function ultra/run/analog_input/有人/Subsystem1/MATLAB Function1 ==
  data: T input; TP output
function TP= fcn(T)
if T<10
    TP=0;
else
    TP=T;
end

== matlab function ultra/run/analog_input/MATLAB Function ==
  data: u input; y output
function y = fcn(u)
if u==9
    y=1;
else
    y=0;
end

== matlab function ultra/run/analog_input/MATLAB Function1 ==
  data: u input; y output; a input
function y = fcn(u,a)
if u==1
    y=15;%%无人规则缓慢转轮
else
    y=a;
end
end

== matlab function ultra/run/analog_input/MATLAB Function3 ==
  data: u input; y output; canok input; workstation input; v input
function y = fcn(u,canok,workstation,v)
if u~=0%%||canok==0
    y=1;
else
    y=0;
end
% if canok==0
%     y=0;
% end
%  if workstation<=0.1
%      y=0;
%  end
%  if v<0.5||v>18
%      y=0;
%  end

== matlab function ultra/run/analog_input/有人/Subsystem1/MATLAB Function ==
  data: v input; T output
function T = fcn(v)
%#codegen
if v<6000*1.88e-3
    T=2100;
elseif v>11000*1.88e-3
    T=800;
else
    T=1100;
end

== matlab function ultra/run/ctrl/Subsystem1/control_strategy/限滑/MPC/MPC/MATLAB Function ==
  data: u input; y output
function y = fcn(u)
if u>=0.169&&u<=0.17
    y=1;
else
    y=0;
end

end

== matlab function ultra/run/ctrl/Subsystem1/control_strategy/限滑/MPC/MPC/MATLAB Function1 ==
  data: u input; y output
function y = fcn(u)
if u>=0.169&&u<=0.17
    y=1;
else
    y=0;
end

end

== matlab function ultra/run/ctrl/Subsystem1/control_strategy/限滑/MPC/MPC/MATLAB Function2 ==
  data: u input; y output
function y = fcn(u)

if u>=0.169&&u<=0.17
    y=1;
else
    y=0;
end

end

== matlab function ultra/run/ctrl/Subsystem1/control_strategy/限滑/MPC/MPC/MATLAB Function3 ==
  data: u input; y output
function y = fcn(u)

if u>=0.169&&u<=0.17
    y=1;
else
    y=0;
end

end

== matlab function ultra/run/ctrl/Subsystem1/control_strategy/MATLAB Function3 ==
  data: y output; angle input
function y = fcn(angle)
if angle>10||angle<-10%4650000,4870000,4741002
    y=1;
else
    y = 0;
end

== matlab function ultra/TX控制器/速度/189左后/MATLAB Function1 ==
  data: v input; T output; a input
function T = fcn(v,a)
% if a>5
%     y = u;
% elseif a>3&&a<5
%     y=1200;
% else
%     y=800;
% end

if v<6000*1.88e-3
    T=2100;
elseif v>11000*1.88e-3
    T=800;
else
    T=1100;
end

== matlab function ultra/RX/lcu——receive/MATLAB Function ==
  data: m input; enable_185 output; enable_185_1 output; enable_188 output; enable_188_1 output; enable_184 output; enable_184_1 output; enable_189 output; enable_189_1 output
%八位无符号数
function [enable_185,enable_185_1,enable_188,enable_188_1,enable_184,enable_184_1,enable_189,enable_189_1] = ErJinZhi(m)
V=zeros(1,8);
a=2;i=8;
while i>0
    V(1,i)=mod(m,a);
    m=fix(m/2);
    i=i-1;
end    
enable_185=V(1,1);%右前
enable_185_1=V(1,2);
enable_188=V(1,3);%右后
enable_188_1=V(1,4);
enable_184=V(1,5);
enable_184_1=V(1,6);%左前
enable_189=V(1,7);
enable_189_1=V(1,8);%左后
end

== matlab function ultra/esc,ABS/MATLAB Function ==
  data: u input; y output
function y = fcn(u)
if u~=0&&u~=9&&u~=2
    y=1;
else
    y=0;
end

== matlab function ultra/run/analog_input/MATLAB Function4 ==
  data: u input; y output; a input
function y = fcn(u,a)
if u==5
    y=0;
else
    y=a;
end
end

== matlab function ultra/RX/工作站/Subsystem3/Subsystem/MATLAB Function ==
  data: u input; y output; CANOK_20 input
function y = fcn(u,CANOK_20)
if CANOK_20==0
    y=0;
else
    y=u;
end

== matlab function ultra/run/analog_input/MATLAB Function5 ==
  data: u input; y output; model input; y6 output
function [y,y6] = fcn(u,model)
if model==8
    y = 0;
    y6=u;
else
    y=u;
    y6=0;
end
if y~=0&&y6~=0
    y=0;
    y6=0;
end
    
end

== matlab function ultra/RX/工作站/Subsystem3/Subsystem/MATLAB Function1 ==
  data: u input; y output; CANOK_20 input
function y = fcn(u,CANOK_20)
% if CANOK_20==0
%     y=0;
% else
    y=u;
% end

== matlab function ultra/无人TX/MATLAB Function1 ==
  data: model input; y output; status input
function y = fcn(model,status)
if (model==1||model==3||model==4||model==6||model==7||model==8)&&(status==3||status==4||status==5)
    y=1;
else
    y=0;
end
if model==8
    y=1;
else
    y=y;
end

== matlab function ultra/无人TX/转向换算/MATLAB Function ==
  data: biaozhi1 output; baocuo input
function biaozhi1  = fcn(baocuo)
persistent i;
     % 初始化状态变量
    if isempty(i)
        i = 1;
    end
    if baocuo==1
        i=1;
    end
    if i>4
        biaozhi1=1;
    else
        biaozhi1=0;       
    end
i=i+1;
end

== matlab function ultra/无人TX/转向换算/Subsystem/MATLAB Function ==
  data: steer output; y output; x input; canok input; baocuo input; k input; d input; rm input; lm input
function [steer,y] = fcn(x,canok,baocuo,k,d,rm,lm)
  persistent i previoussteer;
     % 初始化状态变量
     rm=rm-3000;
     lm=lm+3000;
    if isempty(i)
        i = 0;
    end
    if isempty(previoussteer)
        previoussteer= d;
    end
    if i>0.2     
        steer= k *x+d ;
%         if x==0
%             steer=25092;
%         end
          if steer>rm
              steer=rm;
          end
          if steer<lm
              steer=lm;
          end
    else
        steer=d;
    end
    if canok==0
        steer=previoussteer;
    end
    if baocuo==1
        steer=previoussteer;
    end
    i=i+0.02;
  persistent time  a b;
     % 初始化状态变量
    if isempty(time)
        time = 0;
   
        a=5;
        b=10;
    end
    if baocuo==1
        time=-4;
    end
    if mod(abs(time), 2) == 0
        result = 1;
    else
        result = 0;
    end
    if time<b&&result==0
    y=6;
 
    elseif time<b&&result==1
    y=15;
  
    elseif time>=b
        if result==1
            y=79;
        else
            y=63;
        end
    else
        y=6;
    end   
    time=time+1;
    previoussteer=steer;
%     
%       persistent time1;
%      % 初始化状态变量
%     if isempty(time1)
%         time1 = 0;
%     end
%     if mod(time1, 2) == 0
%         result1 = 1;
%     else
%         result1 = 0;
%     end
%     if time1<2
%     y=6;
%  
%     elseif time1>=2&&time1<4
%     y=15;
%   
%     elseif time1>=4
%         if result1==1
%             y=79;
%         else
%             y=63;
%         end
%     else
%         y=6;
%     end   
%     time1=time1+1;
   
end

== matlab function ultra/RX/工作站/Subsystem3/Subsystem/MATLAB Function2 ==
  data: u input; y output; CANOK_20 input
function y = fcn(u, CANOK_20)


% 初始化位数计数
num_digits = 0; 
% 处理0的情况
if u == 0
    num_digits = 1;
else
    % 计算位数
    num = abs(u);
    while num > 0
        num = floor(num / 10);
        num_digits = num_digits + 1;
    end
end
    divisor = 10 ^ num_digits;
    decimal = u / divisor;
    if u>0
        y=decimal;
    else
        y=-decimal;
    end
    if CANOK_20==0
    y=0;
    end
end

== matlab function ultra/RX/工作站/Subsystem3/Subsystem/MATLAB Function3 ==
  data: u input; y output; CANOK_20 input
function y = fcn(u,CANOK_20)

% 初始化位数计数
num_digits = 0; 
% 处理0的情况
if u == 0
    num_digits = 1;
else
    % 计算位数
    num = abs(u);
    while num > 0
        num = floor(num / 10);
        num_digits = num_digits + 1;
    end
end
    divisor = 10 ^ num_digits;
    decimal = u / divisor;
    if u>0
        y=decimal;
    else
        y=-decimal;
    end
%     if CANOK_20==0
%     y=0;
%     end
end

== matlab function ultra/RX/283 285左前/Subsystem2/Subsystem/MATLAB Function ==
  data: u input; y output
function y = fcn(u)

y = u/594.06;

== matlab function ultra/RX/284 286右前/Subsystem2/Subsystem/MATLAB Function ==
  data: u input; y output
function y = fcn(u)


y = u/594.06;

== matlab function ultra/RX/288 290左后/Subsystem2/Subsystem/MATLAB Function ==
  data: u input; y output
function y = fcn(u)


y = u/594.06;

== matlab function ultra/RX/287 289右后/Subsystem2/Subsystem/MATLAB Function ==
  data: u input; y output
function y = fcn(u)


y = u/594.06;

== matlab function ultra/run/analog_input/无人意图转译/无人/Subsystem1/Desired/MATLAB Function ==
  data: u input; y output
function y = fcn(u)
  % 状态变量
    persistent i
    % 初始化状态变量
    if isempty(i)
       
        i=0;
    end
    y=(u-i)*50;
    if y>23.2
        y=23.2;
    end
    i=u;

== matlab function ultra/run/analog_input/无人意图转译/无人/Subsystem1/Desired/MATLAB Function1 ==
  data: u input; y output
function y = fcn(u)

 persistent i
    % 初始化状态变量
    if isempty(i)
       
        i=0;
    end
    y=(u-i)*50;
    i=u;

== matlab function ultra/TX控制器/扭矩/TEST/MATLAB Function ==
  data: u input; y output
function y = fcn(u)
if u~=0%%&&u~=6
    y=1;
else
    y=0;
end

== matlab function ultra/TX控制器/MATLAB Function ==
  data: u input; ysudu output; yniuju output; model input; v input
function [ysudu,yniuju] = fcn(u,model,v)
if u>25
    yniuju=1;
    ysudu=0;
else
    yniuju=0;
    ysudu=1;
end

if v<0.5||v>18
     yniuju=0;
     ysudu=1;
end
if model==9
    yniuju=1;
    ysudu=0;
end
if model==0
    yniuju=1;
    ysudu=0;
end
if yniuju==ysudu
    yniuju=0;
    ysudu=0;
end

== matlab function ultra/run/kalman_filter ==
  data: a_k_1 input; y output; v_k_1 input; v_k input; V_MIN input
function y = fcn(a_k_1,v_k_1,v_k,V_MIN)
A=1;
H=1;
% x_real=v_k_1+0.02*a_k_1;%首先给出一个相应的估计值
% z=0;
% w=0;
% v=0;
% %%噪声信号
%     w=1*randn;
%     v=1*randn;
% %%状态方程
%     x_real=A*v_k_1+0.02*a_k_1+w;
% %%观测方程
%     z=H*x_real+v;
% persistent xhat;
%      % 初始化状态变量
%     if isempty(xhat)
%         xhat = V_MIN;
%     end

    z=H*v_k;
%%kalman_filter  根据上述得观测值来不断更新  
xhat=v_k;
xhat=v_k_1+0.02*a_k_1;%先验估计
Q=1;
R=0.01;
Pk=1;
Pk_bar=0;%先验协方差

    xhat_=v_k_1+0.02*a_k_1;%先验估计
    Pk_bar=A*Pk*A'+Q;
    Kk=Pk_bar*H'/(H*Pk_bar*H'+R);
    xhat= xhat_+ Kk*(z-H* xhat_);%最优估计值
    Pk=(1-Kk*H)*Pk_bar;
if v_k<0.1
    y=V_MIN;%即转轮时不使用惯导信息
elseif abs(xhat-v_k)>0.5
    y=v_k;
else
    y = xhat;
end
end

== matlab function ultra/RX/转向——receive编码器/Subsystem3/Subsystem/MATLAB Function ==
  data: u input; y output
function y = fcn(u)
if u<180
    y=-u/4.1;
else
    y=(360-u)/4.1;
end

== matlab function ultra/无人TX/转向换算/Subsystem/转向修正 ==
  data: steerbianmaqi input; steerangle input; steernew output; steer input; error output; k input; KP input; KI input; KD input; model input
function [steernew,error]  = carPIDWithSlipControl(steerbianmaqi,steerangle,steer,k,KP,KI,KD,model)
    % 赛车PID控制器参数
    if k==0
%         kp=1.25;
%         ki=0.27;
%         kd=0.6;
%         kp = 1.5;
%         ki = 0.4;
%         kd = 0.65;
%    kp = 1.2;
%     ki = 0.25;
%     kd = 0.55;
        kp = 0.4;
        ki = 0.13;
        kd = 0.3;
     else
        kp=KP;
        ki=KI;
        kd=KD;
    end
    if (model==1)&&(steer<5)
        kp=0.8;
        ki=0.1;
        kd=0.15;
    end
%     else
%         kp=KP;
%         ki=KI;
%         kd=KD;
%     end
    %kp = 1.2;
    %ki = 0.25;
    %kd = 0.55;
    % 状态变量
    persistent integral previous_error  presteer preerrorbianmaqi
    
    % 初始化状态变量
    if isempty(integral)
        integral = 0;
        previous_error = 0;
       presteer=0;
        preerrorbianmaqi=0;
    end
    errorbianmaqi=steerangle-steerbianmaqi;
    % PID控制器计算
    error = steer - steerbianmaqi;
    integral = integral + error*0.02;
    derivative = (error - previous_error)/0.02;
    

%     if abs(steer)<0.5%零点消除抖震
%         kp=0;
%         ki=0;
%         kd=0;
%     end
        
   
    K= kp * error + ki * integral + kd * derivative;
   if K<0.05%消抖
       K=0;
   end
    
        steernew =steer+K;

    if (steer*presteer<0)
        integral=0;
        if (abs(error)>1.3)&&(abs(steer)<5)&&(abs(steer-steerbianmaqi)>3)&&(model==1)
            if steer>0
                steernew=7;
            end
            if steer<0
                steernew=-7;
            end
        end
    end
    % 保存上一个误差用于下次计算
    previous_error = error;
     preerrorbianmaqi= errorbianmaqi;
     presteer=steer;
end

== matlab function ultra/TOWORKSTATION/转向/MATLAB Function ==
  data: u input; y output
function y = fcn(u)
if u==9
    y=1;
else
    y=0;
end

== matlab function ultra/TOWORKSTATION/转向/Subsystem/MATLAB Function ==
  data: biaozhi1 output
function biaozhi1  = fcn
persistent i;
     % 初始化状态变量
    if isempty(i)
        i = 1;
    end
    if i>16
        biaozhi1=1;
    else
        biaozhi1=0;
    end
    i=i+1;
end

== matlab function ultra/run/analog_input/无人意图转译/无人/Subsystem1/MATLAB Function ==
  data: u input; y output; u2 input
function y = fcn(u,u2)

y = u-u2;

== matlab function ultra/run/analog_input/无人意图转译/无人/Subsystem1/Desired/MATLAB Function2 ==
  data: u1 input; y output; u2 input; u3 input; u4 input; u5 input; model input; v1 input; v2 input; v3 input; v4 input; v5 input; V output
function [y,V] = fcn(u1,u2,u3,u4,u5,model,v1,v2,v3,v4,v5)
y=u1;
V=v1;
if u1>5&&u1<=10
    y=(u1+u2+u3)/3;
    V=(v1+v2+v3)/3;
end
if u1>10
    y=(u1+u2+u3+u4+u5)/5;
    V=(v1+v2+v3+v4+v5)/5;
end
if model==1
    y=u1;
    V=v1;
end
if model==0
    y=0;
    V=0;
end
if u1<0
    y=u1;
    V=v1;
end

== matlab function ultra/run/ctrl/Subsystem1/control_strategy/限滑/MATLAB Function ==
  data: slip_ratio_front_left input; torque_front_left output; slip_ratio_front_right input; slip_ratio_rear_left input; slip_ratio_rear_right input; e_prev input; dt input; torque_front_right output; torque_rear_left output; torque_rear_right output
function [torque_front_left, torque_front_right, torque_rear_left, torque_rear_right] = SlipRatioControl(slip_ratio_front_left, slip_ratio_front_right, slip_ratio_rear_left, slip_ratio_rear_right,  e_prev, dt)

% 参数设定
lambda = 5; % 调整因子，用于滑模面设计，实际应用中可能需要调整
boundary_thickness = 0.1; % 边界层厚度，用于sigmoid函数，以确保输出在合理范围内
max_torque = 2000; % 最大扭矩，表示车辆能够输出的最大扭矩
slip_ratio_desired=0.2;
% 内部函数，为每个轮子计算扭矩
function torque = computeTorque(slip_ratio_actual, e_prev)
    % 计算误差及其导数
    e = slip_ratio_desired - slip_ratio_actual;
    e_dot = (e - e_prev) / dt;
    
    % 滑模控制
    s = e_dot + lambda * e;
    
    % 使用软饱和函数（sigmoid函数）计算扭矩指令
    torque = max_torque / (1 + exp(-10 * (s - boundary_thickness)));
    
    % 限制扭矩值
    torque = min(max_torque, torque);
end

% 为每个轮子计算扭矩
torque_front_left = computeTorque(slip_ratio_front_left, e_prev(1));
torque_front_right = computeTorque(slip_ratio_front_right, e_prev(2));
torque_rear_left = computeTorque(slip_ratio_rear_left, e_prev(3));
torque_rear_right = computeTorque(slip_ratio_rear_right, e_prev(4));

% 更新上一次的误差
e_prev(1) = slip_ratio_desired - slip_ratio_front_left;
e_prev(2) = slip_ratio_desired - slip_ratio_front_right;
e_prev(3) = slip_ratio_desired - slip_ratio_rear_left;
e_prev(4) = slip_ratio_desired - slip_ratio_rear_right;

end

== matlab function ultra/RX/lcu——receive/Subsystem1/Subsystem/MATLAB Function2 ==
  data: u input; y output
function y = fcn(u)
% if(u==1||u==4)
if(u==4)
    y=1;
else
    y=0;
end

== matlab function ultra/RX/工作站/Subsystem3/Subsystem/MATLAB Function4 ==
  data: u input; y output; nengbunengpao input; model input
function y = fcn(u,nengbunengpao,model)
if nengbunengpao==1
    y = u;
else
    y=0;
end
if model==6
    y=u;
else
    y=y;
end

== matlab function ultra/run/MATLAB Function1 ==
  data: V_lon input; V_longitudinal output; V_lat input; theta_deg input; V_lateral output; V_MIN input
function [V_longitudinal, V_lateral] = calculateVelocities(V_lon, V_lat, theta_deg,V_MIN)
    % 将角度转换为弧度
    theta_rad = deg2rad(theta_deg);

    % 计算纵向速度和横向速度
    V_longitudinal_ = V_lon * sin(theta_rad) + V_lat * cos(theta_rad);
    if V_longitudinal_<0.2
         V_longitudinal=V_MIN;
    else
         V_longitudinal= V_longitudinal_;
    end
    V_lateral = V_lon * cos(theta_rad) -V_lat * sin(theta_rad);
end

== matlab function ultra/run/ctrl/Subsystem1/control_strategy/滑模控制 ==
  data: slip_ratio_fl input; slip_ratio_fr input; slip_ratio_rl input; slip_ratio_rr input; torque_cmd_fl output; driver_torque_cmd_fl input; driver_torque_cmd_fr input; driver_torque_cmd_rl input; driver_torque_cmd_rr input; torque_cmd_fr output; torque_cmd_rl output; torque_cmd_rr output
function [torque_cmd_fl, torque_cmd_fr, torque_cmd_rl, torque_cmd_rr] = SlipRatioControl(slip_ratio_fl, slip_ratio_fr, slip_ratio_rl, slip_ratio_rr,   driver_torque_cmd_fl, driver_torque_cmd_fr, driver_torque_cmd_rl, driver_torque_cmd_rr)

    % 每个轮都有自己的误差历史记录
    persistent e_prev_fl e_prev_fr e_prev_rl e_prev_rr i driver_weight
    if isempty(e_prev_fl)
        e_prev_fl = 0; e_prev_fr = 0; e_prev_rl = 0; e_prev_rr = 0;
        driver_weight = 0.5;  % 车手命令的权重
        i=0;
    end

    % 设定参数
    lambda = 3;            % 滑模面设计参数
    K = 0.5;               % 滑模增益
    delta = 0.05;          % 滑模边界，小于此值时不做扭矩调整
%     driver_weight = 0.05;  % 车手命令的权重
    desired_slip_ratio=0.2;
    % 定义一个内部函数来进行滑膜控制，这样可以为每个轮重复使用
    function [torque_cmd, e_prev,e] = singleWheelControl(slip_ratio, desired_slip_ratio, driver_torque_cmd, e_prev)
        % 计算误差和误差的变化率
        e = desired_slip_ratio - slip_ratio;
        e_dot = (e - e_prev) / 0.02;
        s = e_dot + lambda * e;

        % 滑模控制策略
        if abs(s) < delta
            torque_adjustment = 0;  % s小于滑模边界时不做调整
        else
            torque_adjustment = K * s;  % 根据s的符号进行扭矩调整
        end

        % 结合车手的扭矩命令，并应用滑模控制的调整
        torque_cmd = driver_torque_cmd + driver_weight * driver_torque_cmd * torque_adjustment;
        torque_cmd = max(0, torque_cmd);  % 保证扭矩命令为正
        torque_cmd = min(2000, torque_cmd);  % 保证扭矩小于2000

        % 更新误差
        e_prev = e;
    end
    % 对每个轮应用滑模控制策略
    [torque_cmd_fl, e_prev_fl,efl] = singleWheelControl(slip_ratio_fl, desired_slip_ratio, driver_torque_cmd_fl, e_prev_fl);
    [torque_cmd_fr, e_prev_fr,efr] = singleWheelControl(slip_ratio_fr, desired_slip_ratio, driver_torque_cmd_fr, e_prev_fr);
    [torque_cmd_rl, e_prev_rl,erl] = singleWheelControl(slip_ratio_rl, desired_slip_ratio, driver_torque_cmd_rl, e_prev_rl);
    [torque_cmd_rr, e_prev_rr,err] = singleWheelControl(slip_ratio_rr, desired_slip_ratio, driver_torque_cmd_rr, e_prev_rr);
     %安全程序
     if (efl>0.8||efr>0.8||erl>0.8||err>0.8)
         i=i+1;
         if i>100
             driver_weight=0;
         end
     end
     if (efl<0.3&&efr<0.3&&erl<0.3&&err<0.3)
         i=0;
     end

end
